simulink model "ArduCopter_3DR"  (R2016b)
settings: Solver=ode45  StartTime=0.0  StopTime=10.0  RelTol=1e-3  EnableMultiTasking=on
undefined symbols (not defined in the file): i_max, i_min, Jm, k_thrust, k_torque, L, R, v_max, v_min
settings Model: Creator=pa872d  LastModifiedBy=aaronniemiec
settings DataIOCC: LimitDataPoints=on  SaveFormat=Array
settings OptimizationCC: LifeSpan=inf
settings DebuggingCC: SFUnexpectedBacktrackingDiag=warning  SFNoUnconditionalDefaultTransitionDiag=warning  SFExecutionAtInitializationDiag=none
settings HardwareCC: ProdBitPerPointer=32  ProdBitPerSizeT=32  ProdBitPerPtrDiffT=32  ProdLargestAtomicFloat=None  ProdIntDivRoundTo=Undefined  ProdEndianess=Unspecified  ProdWordSize=32  ProdHWDeviceType=32-bit Generic
settings ModelReferenceCC: PropagateSignalLabelsOutOfModel=off
settings GRTTargetCC: TargetLangStandard=C89/C90 (ANSI)  GeneratePreprocessorConditionals=Disable all
settings ConfigComp: CovMetricSettings=dw  CovHtmlReporting=on  CovSaveCumulativeToWorkspaceVar=on  CovSaveSingleToWorkspaceVar=on  CovExternalEMLEnable=off

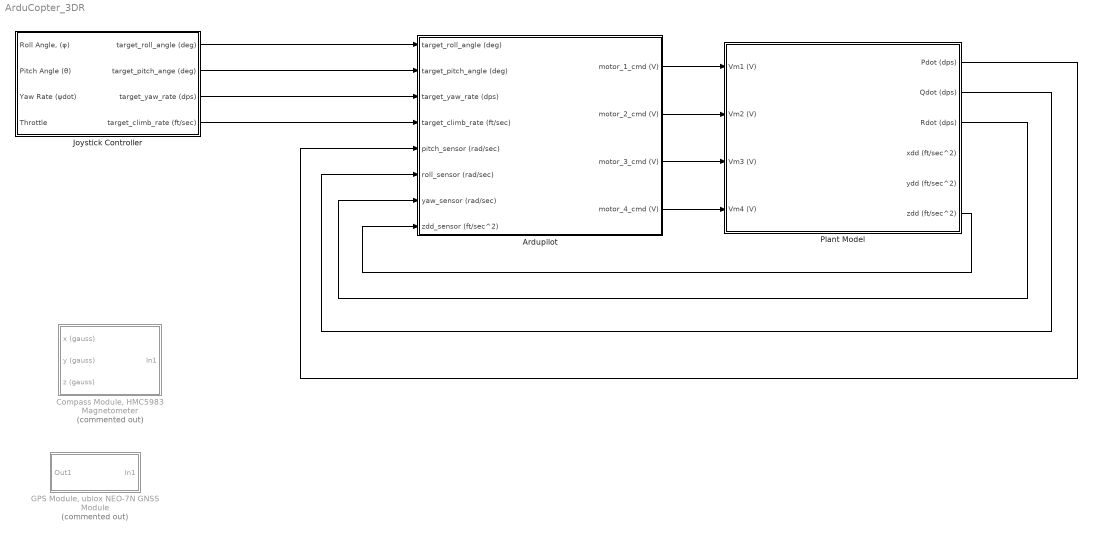
== system ArduCopter_3DR ==
  Ardupilot : Subsystem
  "Compass Module, HMC5983 Magnetometer" : Subsystem  Commented=on
  "GPS Module, ublox NEO-7N GNSS Module" : Subsystem  Commented=on
  Joystick Controller : Subsystem
  Plant Model : Subsystem
  wires:
  Joystick Controller/1(target_roll_angle (deg)) -> Ardupilot/1(target_roll_angle (deg))
  Joystick Controller/2(target_pitch_ange (deg)) -> Ardupilot/2(target_pitch_angle (deg))
  Joystick Controller/3(target_yaw_rate (dps)) -> Ardupilot/3(target_yaw_rate (dps))
  Joystick Controller/4(target_climb_rate (ft/sec)) -> Ardupilot/4(target_climb_rate (ft/sec))
  Plant Model/1(Pdot (dps)) -> Ardupilot/5(pitch_sensor (rad/sec))
  Plant Model/3(Rdot (dps)) -> Ardupilot/7(yaw_sensor (rad/sec))
  Ardupilot/1(motor_1_cmd (V)) -> Plant Model/1(Vm1 (V))
  Ardupilot/2(motor_2_cmd (V)) -> Plant Model/2(Vm2 (V))
  Ardupilot/3(motor_3_cmd (V)) -> Plant Model/3(Vm3 (V))
  Ardupilot/4(motor_4_cmd (V)) -> Plant Model/4(Vm4 (V))
  Plant Model/2(Qdot (dps)) -> Ardupilot/6(roll_sensor (rad/sec))
  Plant Model/6(zdd (ft/sec^2)) -> Ardupilot/8(zdd_sensor (ft/sec^2))

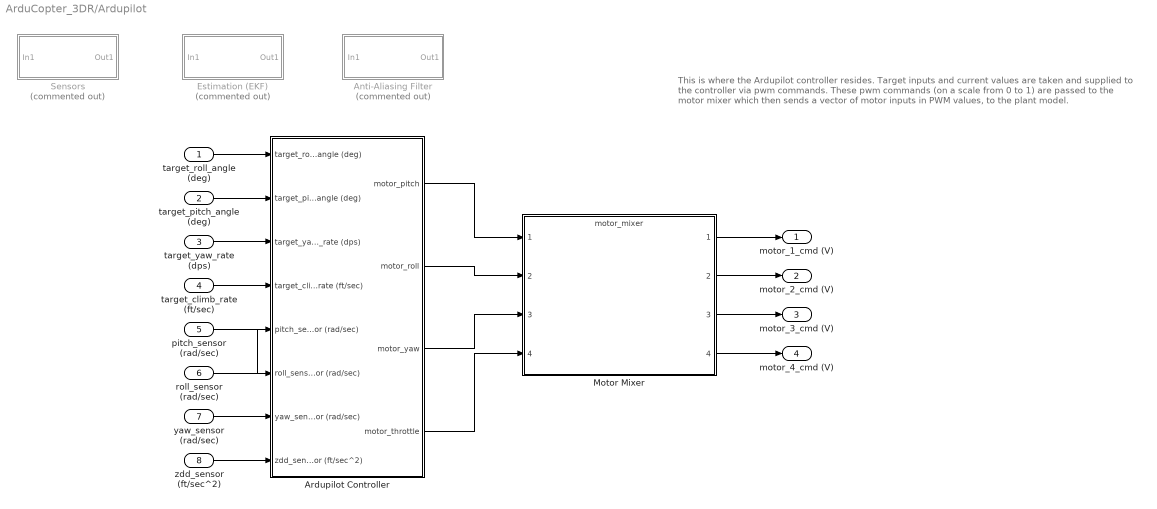
== system ArduCopter_3DR/Ardupilot ==
  note: This is where the Ardupilot controller resides. Target inputs and current values are taken and
      | supplied to the controller via pwm commands. These pwm commands (on a scale from 0 to 1) are passed to the motor mixer which then
      | sends a vector of motor inputs in PWM values, to the plant model.
  target_roll_angle (deg) : Inport
  target_pitch_angle (deg) : Inport  Port=2
  target_yaw_rate (dps) : Inport  Port=3
  target_climb_rate (ft/sec) : Inport  Port=4
  pitch_sensor (rad/sec) : Inport  Port=5
  roll_sensor (rad/sec) : Inport  Port=6
  yaw_sensor (rad/sec) : Inport  Port=7
  zdd_sensor (ft/sec^2) : Inport  Port=8
  Anti-Aliasing Filter : Subsystem  Commented=on
  Ardupilot Controller : Subsystem
  Estimation (EKF) : Subsystem  Commented=on
  Motor Mixer : ModelReference  ModelNameDialog=motor_mixer.slx  SimulationMode=Normal  ModelReferenceVersion=1.6
  Sensors : Subsystem  Commented=on
  motor_1_cmd (V) : Outport
  motor_2_cmd (V) : Outport  Port=2
  motor_3_cmd (V) : Outport  Port=3
  motor_4_cmd (V) : Outport  Port=4
  wires:
  Motor Mixer/2 -> motor_2_cmd (V)/1
  Motor Mixer/4 -> motor_4_cmd (V)/1
  Motor Mixer/3 -> motor_3_cmd (V)/1
  target_roll_angle (deg)/1 -> Ardupilot Controller/1(target_roll_angle (deg))
  target_pitch_angle (deg)/1 -> Ardupilot Controller/2(target_pitch_angle (deg))
  target_yaw_rate (dps)/1 -> Ardupilot Controller/3(target_yaw_rate (dps))
  target_climb_rate (ft/sec)/1 -> Ardupilot Controller/4(target_climb_rate (ft/sec))
  Motor Mixer/1 -> motor_1_cmd (V)/1
  yaw_sensor (rad/sec)/1 -> Ardupilot Controller/7(yaw_sensor (rad/sec))
  zdd_sensor (ft/sec^2)/1 -> Ardupilot Controller/8(zdd_sensor (ft/sec^2))
  pitch_sensor (rad/sec)/1 -> Ardupilot Controller/6(roll_sensor (rad/sec))
  roll_sensor (rad/sec)/1 -> Ardupilot Controller/5(pitch_sensor (rad/sec))
  Ardupilot Controller/1(motor_pitch) -> Motor Mixer/1
  Ardupilot Controller/2(motor_roll) -> Motor Mixer/2
  Ardupilot Controller/3(motor_yaw) -> Motor Mixer/3
  Ardupilot Controller/4(motor_throttle) -> Motor Mixer/4

== system ArduCopter_3DR/Compass Module, HMC5983 Magnetometer ==
  In1 : Inport
  x (gauss) : Outport
  y (gauss) : Outport  Port=2
  z (gauss) : Outport  Port=3

== system ArduCopter_3DR/GPS Module, ublox NEO-7N GNSS Module ==
  In1 : Inport
  Out1 : Outport
  wires:
  In1/1 -> Out1/1

== system ArduCopter_3DR/Joystick Controller ==
  "Roll Angle, (φ)" : Inport
  Pitch Angle (θ) : Inport  Port=2
  Yaw Rate (ψdot) : Inport  Port=3
  Throttle : Inport  Port=4
  target_roll_angle (deg) : Outport
  target_pitch_ange (deg) : Outport  Port=2
  target_yaw_rate (dps) : Outport  Port=3
  target_climb_rate (ft/sec) : Outport  Port=4
  wires:
  Yaw Rate (ψdot)/1 -> target_yaw_rate (dps)/1
  Throttle/1 -> target_climb_rate (ft/sec)/1
  Pitch Angle (θ)/1 -> target_pitch_ange (deg)/1
  "Roll Angle, (φ)"/1 -> target_roll_angle (deg)/1

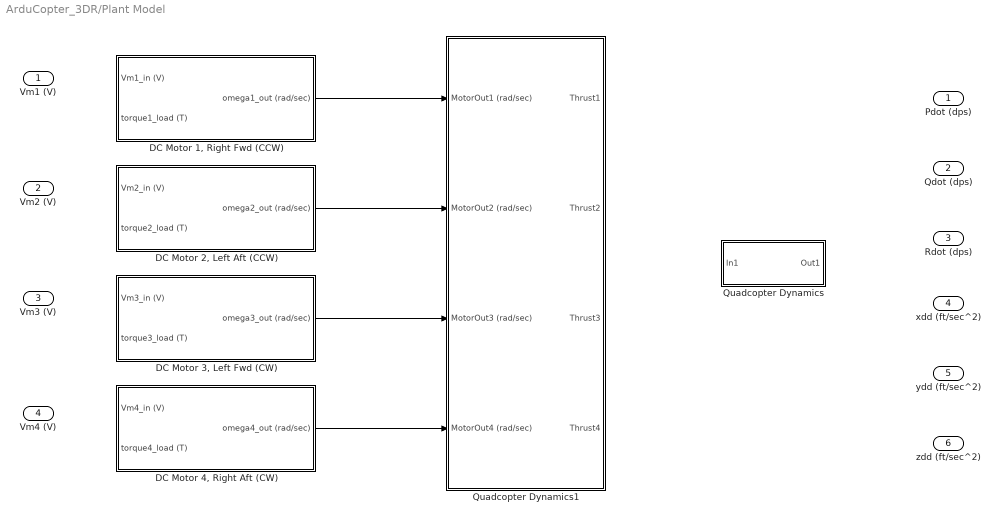
== system ArduCopter_3DR/Plant Model ==
  Vm1 (V) : Inport
  Vm2 (V) : Inport  Port=2
  Vm3 (V) : Inport  Port=3
  Vm4 (V) : Inport  Port=4
  "DC Motor 1, Right Fwd (CCW)" : Subsystem
  "DC Motor 2, Left Aft (CCW)" : Subsystem
  "DC Motor 3, Left Fwd (CW)" : Subsystem
  "DC Motor 4, Right Aft (CW)" : Subsystem
  Quadcopter Dynamics : Subsystem
  Quadcopter Dynamics1 : Subsystem
  Pdot (dps) : Outport
  Qdot (dps) : Outport  Port=2
  Rdot (dps) : Outport  Port=3
  xdd (ft/sec^2) : Outport  Port=4
  ydd (ft/sec^2) : Outport  Port=5
  zdd (ft/sec^2) : Outport  Port=6
  wires:
  "DC Motor 1, Right Fwd (CCW)"/1(omega1_out (rad/sec)) -> Quadcopter Dynamics1/1(MotorOut1 (rad/sec))
  "DC Motor 2, Left Aft (CCW)"/1(omega2_out (rad/sec)) -> Quadcopter Dynamics1/2(MotorOut2 (rad/sec))
  "DC Motor 3, Left Fwd (CW)"/1(omega3_out (rad/sec)) -> Quadcopter Dynamics1/3(MotorOut3 (rad/sec))
  "DC Motor 4, Right Aft (CW)"/1(omega4_out (rad/sec)) -> Quadcopter Dynamics1/4("MotorOut4 (rad/sec) ")

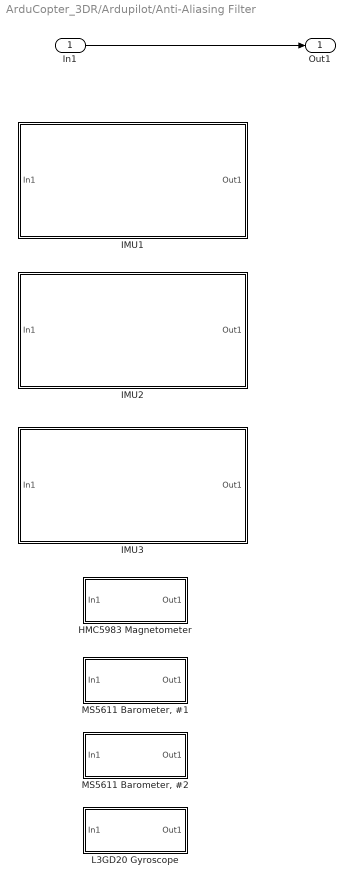
== system ArduCopter_3DR/Ardupilot/Anti-Aliasing Filter ==
  In1 : Inport
  HMC5983 Magnetometer : Subsystem
  IMU1 : Subsystem
  IMU2 : Subsystem
  IMU3 : Subsystem
  L3GD20 Gyroscope : Subsystem
  "MS5611 Barometer, #1" : Subsystem
  "MS5611 Barometer, #2" : Subsystem
  Out1 : Outport
  wires:
  In1/1 -> Out1/1

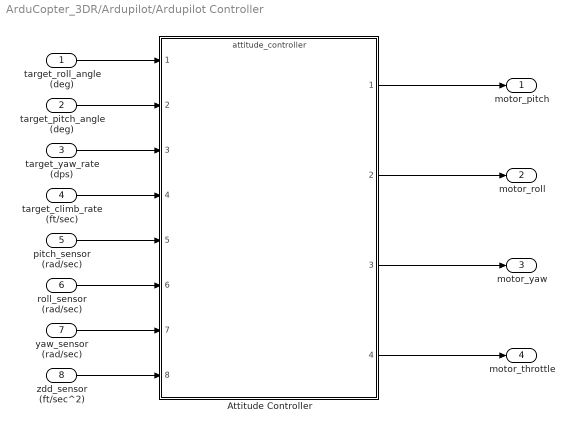
== system ArduCopter_3DR/Ardupilot/Ardupilot Controller ==
  target_roll_angle (deg) : Inport
  target_pitch_angle (deg) : Inport  Port=2
  target_yaw_rate (dps) : Inport  Port=3
  target_climb_rate (ft/sec) : Inport  Port=4
  pitch_sensor (rad/sec) : Inport  Port=5
  roll_sensor (rad/sec) : Inport  Port=6
  yaw_sensor (rad/sec) : Inport  Port=7
  zdd_sensor (ft/sec^2) : Inport  Port=8
  Attitude Controller : ModelReference  ModelNameDialog=attitude_controller.slx  SimulationMode=Normal  ModelReferenceVersion=1.15
  motor_pitch : Outport
  motor_roll : Outport  Port=2
  motor_yaw : Outport  Port=3
  motor_throttle : Outport  Port=4
  wires:
  Attitude Controller/4 -> motor_throttle/1
  Attitude Controller/3 -> motor_yaw/1
  target_roll_angle (deg)/1 -> Attitude Controller/1
  target_pitch_angle (deg)/1 -> Attitude Controller/2
  target_yaw_rate (dps)/1 -> Attitude Controller/3
  target_climb_rate (ft/sec)/1 -> Attitude Controller/4
  yaw_sensor (rad/sec)/1 -> Attitude Controller/7
  zdd_sensor (ft/sec^2)/1 -> Attitude Controller/8
  roll_sensor (rad/sec)/1 -> Attitude Controller/6
  pitch_sensor (rad/sec)/1 -> Attitude Controller/5
  Attitude Controller/2 -> motor_roll/1
  Attitude Controller/1 -> motor_pitch/1

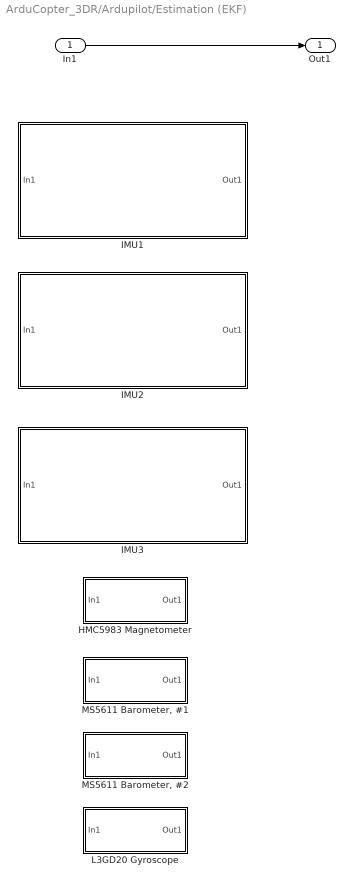
== system ArduCopter_3DR/Ardupilot/Estimation (EKF) ==
  In1 : Inport
  HMC5983 Magnetometer : Subsystem
  IMU1 : Subsystem
  IMU2 : Subsystem
  IMU3 : Subsystem
  L3GD20 Gyroscope : Subsystem
  "MS5611 Barometer, #1" : Subsystem
  "MS5611 Barometer, #2" : Subsystem
  Out1 : Outport
  wires:
  In1/1 -> Out1/1

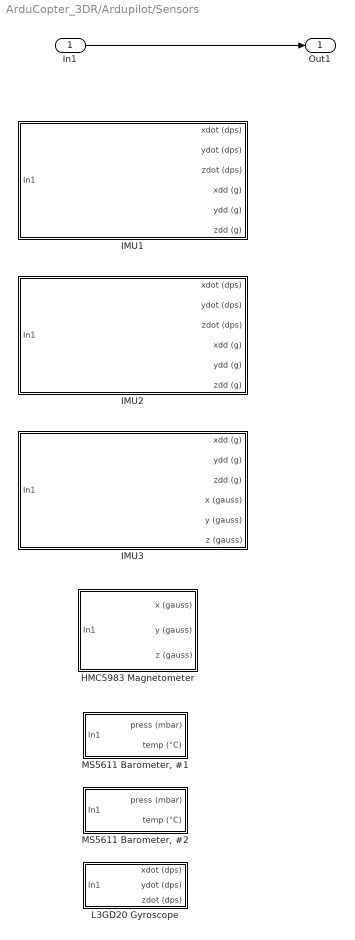
== system ArduCopter_3DR/Ardupilot/Sensors ==
  In1 : Inport
  HMC5983 Magnetometer : Subsystem
  IMU1 : Subsystem
  IMU2 : Subsystem
  IMU3 : Subsystem
  L3GD20 Gyroscope : Subsystem
  "MS5611 Barometer, #1" : Subsystem
  "MS5611 Barometer, #2" : Subsystem
  Out1 : Outport
  wires:
  In1/1 -> Out1/1

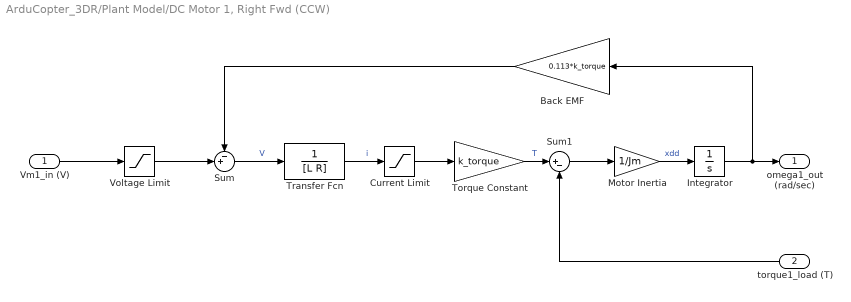
== system ArduCopter_3DR/Plant Model/DC Motor 1, Right Fwd (CCW) ==
  Vm1_in (V) : Inport
  torque1_load (T) : Inport  Port=2
  Back EMF : Gain  Gain=0.113*k_torque
  Current Limit : Saturate  UpperLimit=i_max  LowerLimit=i_min
  Integrator : Integrator
  Motor Inertia : Gain  Gain=1/Jm
  Sum : Sum  Inputs=-+|
  Sum1 : Sum  Inputs=|+-
  Torque Constant : Gain  Gain=k_torque
  Transfer Fcn : TransferFcn  Denominator=[L R]
  Voltage Limit : Saturate  UpperLimit=v_max  LowerLimit=v_min
  omega1_out (rad/sec) : Outport
  wires:
  Vm1_in (V)/1 -> Voltage Limit/1
  Voltage Limit/1 -> Sum/2
  torque1_load (T)/1 -> Sum1/2
  Sum1/1 -> Motor Inertia/1
  Integrator/1 -> omega1_out (rad/sec)/1, Back EMF/1
  Motor Inertia/1 -> Integrator/1  "xdd"
  Back EMF/1 -> Sum/1
  Torque Constant/1 -> Sum1/1  "T"
  Current Limit/1 -> Torque Constant/1
  Sum/1 -> Transfer Fcn/1  "V"
  Transfer Fcn/1 -> Current Limit/1  "i"

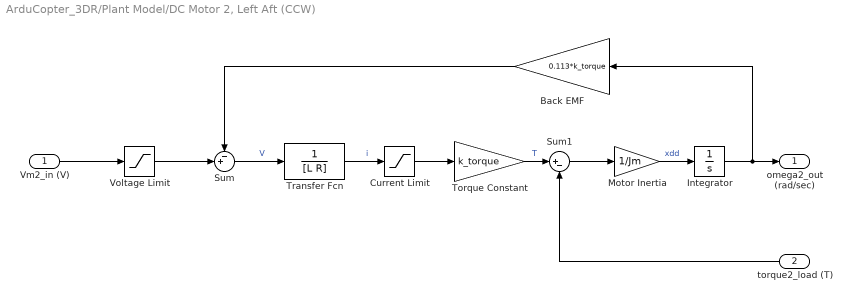
== system ArduCopter_3DR/Plant Model/DC Motor 2, Left Aft (CCW) ==
  Vm2_in (V) : Inport
  torque2_load (T) : Inport  Port=2
  Back EMF : Gain  Gain=0.113*k_torque
  Current Limit : Saturate  UpperLimit=i_max  LowerLimit=i_min
  Integrator : Integrator
  Motor Inertia : Gain  Gain=1/Jm
  Sum : Sum  Inputs=-+|
  Sum1 : Sum  Inputs=|+-
  Torque Constant : Gain  Gain=k_torque
  Transfer Fcn : TransferFcn  Denominator=[L R]
  Voltage Limit : Saturate  UpperLimit=v_max  LowerLimit=v_min
  omega2_out (rad/sec) : Outport
  wires:
  Vm2_in (V)/1 -> Voltage Limit/1
  Voltage Limit/1 -> Sum/2
  torque2_load (T)/1 -> Sum1/2
  Sum1/1 -> Motor Inertia/1
  Integrator/1 -> omega2_out (rad/sec)/1, Back EMF/1
  Motor Inertia/1 -> Integrator/1  "xdd"
  Back EMF/1 -> Sum/1
  Torque Constant/1 -> Sum1/1  "T"
  Current Limit/1 -> Torque Constant/1
  Sum/1 -> Transfer Fcn/1  "V"
  Transfer Fcn/1 -> Current Limit/1  "i"

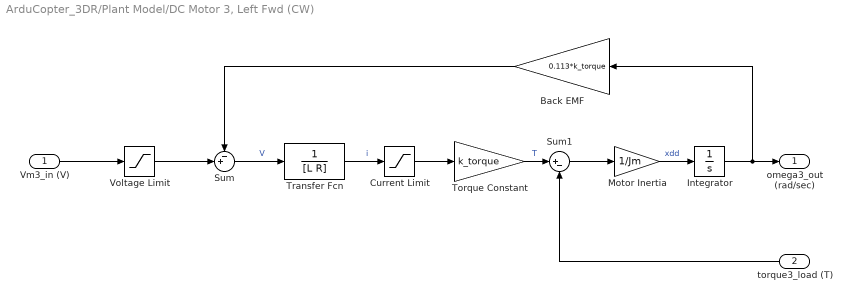
== system ArduCopter_3DR/Plant Model/DC Motor 3, Left Fwd (CW) ==
  Vm3_in (V) : Inport
  torque3_load (T) : Inport  Port=2
  Back EMF : Gain  Gain=0.113*k_torque
  Current Limit : Saturate  UpperLimit=i_max  LowerLimit=i_min
  Integrator : Integrator
  Motor Inertia : Gain  Gain=1/Jm
  Sum : Sum  Inputs=-+|
  Sum1 : Sum  Inputs=|+-
  Torque Constant : Gain  Gain=k_torque
  Transfer Fcn : TransferFcn  Denominator=[L R]
  Voltage Limit : Saturate  UpperLimit=v_max  LowerLimit=v_min
  omega3_out (rad/sec) : Outport
  wires:
  Vm3_in (V)/1 -> Voltage Limit/1
  Voltage Limit/1 -> Sum/2
  torque3_load (T)/1 -> Sum1/2
  Sum1/1 -> Motor Inertia/1
  Integrator/1 -> omega3_out (rad/sec)/1, Back EMF/1
  Motor Inertia/1 -> Integrator/1  "xdd"
  Back EMF/1 -> Sum/1
  Torque Constant/1 -> Sum1/1  "T"
  Current Limit/1 -> Torque Constant/1
  Sum/1 -> Transfer Fcn/1  "V"
  Transfer Fcn/1 -> Current Limit/1  "i"

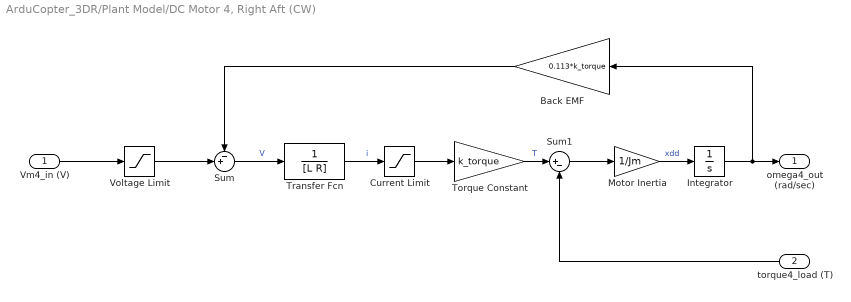
== system ArduCopter_3DR/Plant Model/DC Motor 4, Right Aft (CW) ==
  Vm4_in (V) : Inport
  torque4_load (T) : Inport  Port=2
  Back EMF : Gain  Gain=0.113*k_torque
  Current Limit : Saturate  UpperLimit=i_max  LowerLimit=i_min
  Integrator : Integrator
  Motor Inertia : Gain  Gain=1/Jm
  Sum : Sum  Inputs=-+|
  Sum1 : Sum  Inputs=|+-
  Torque Constant : Gain  Gain=k_torque
  Transfer Fcn : TransferFcn  Denominator=[L R]
  Voltage Limit : Saturate  UpperLimit=v_max  LowerLimit=v_min
  omega4_out (rad/sec) : Outport
  wires:
  Vm4_in (V)/1 -> Voltage Limit/1
  Voltage Limit/1 -> Sum/2
  torque4_load (T)/1 -> Sum1/2
  Sum1/1 -> Motor Inertia/1
  Integrator/1 -> omega4_out (rad/sec)/1, Back EMF/1
  Motor Inertia/1 -> Integrator/1  "xdd"
  Back EMF/1 -> Sum/1
  Torque Constant/1 -> Sum1/1  "T"
  Current Limit/1 -> Torque Constant/1
  Sum/1 -> Transfer Fcn/1  "V"
  Transfer Fcn/1 -> Current Limit/1  "i"

== system ArduCopter_3DR/Plant Model/Quadcopter Dynamics ==
  In1 : Inport
  Out1 : Outport
  wires:
  In1/1 -> Out1/1

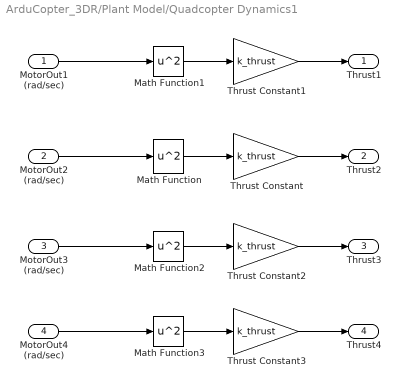
== system ArduCopter_3DR/Plant Model/Quadcopter Dynamics1 ==
  MotorOut1 (rad/sec) : Inport
  MotorOut2 (rad/sec) : Inport  Port=2
  MotorOut3 (rad/sec) : Inport  Port=3
  "MotorOut4 (rad/sec) " : Inport  Port=4
  Math Function{,1..3} (4 alike) : Math  Operator=square  SaturateOnIntegerOverflow=on
  Thrust Constant{,1..3} (4 alike) : Gain  Gain=k_thrust
  Thrust1 : Outport
  Thrust2 : Outport  Port=2
  Thrust3 : Outport  Port=3
  Thrust4 : Outport  Port=4
  wires:
  MotorOut2 (rad/sec)/1 -> Math Function/1
  Math Function/1 -> Thrust Constant/1
  Thrust Constant/1 -> Thrust2/1
  MotorOut1 (rad/sec)/1 -> Math Function1/1
  Math Function1/1 -> Thrust Constant1/1
  Thrust Constant1/1 -> Thrust1/1
  MotorOut3 (rad/sec)/1 -> Math Function2/1
  Math Function2/1 -> Thrust Constant2/1
  Thrust Constant2/1 -> Thrust3/1
  "MotorOut4 (rad/sec) "/1 -> Math Function3/1
  Math Function3/1 -> Thrust Constant3/1
  Thrust Constant3/1 -> Thrust4/1

== system ArduCopter_3DR/Ardupilot/Anti-Aliasing Filter/HMC5983 Magnetometer ==
  In1 : Inport
  Out1 : Outport
  wires:
  In1/1 -> Out1/1

== system ArduCopter_3DR/Ardupilot/Anti-Aliasing Filter/IMU1 ==
  In1 : Inport
  MPU6000 Accelerometer : Subsystem
  MPU6000 Gyroscope : Subsystem
  Out1 : Outport
  wires:
  In1/1 -> Out1/1

== system ArduCopter_3DR/Ardupilot/Anti-Aliasing Filter/IMU2 ==
  In1 : Inport
  MPU6000 Accelerometer : Subsystem
  MPU6000 Gyroscope : Subsystem
  Out1 : Outport
  wires:
  In1/1 -> Out1/1

== system ArduCopter_3DR/Ardupilot/Anti-Aliasing Filter/IMU3 ==
  In1 : Inport
  LSM303D Accelerometer : Subsystem
  LSM303D Magnetometer : Subsystem
  Out1 : Outport
  wires:
  In1/1 -> Out1/1

== system ArduCopter_3DR/Ardupilot/Anti-Aliasing Filter/L3GD20 Gyroscope ==
  In1 : Inport
  Out1 : Outport
  wires:
  In1/1 -> Out1/1

== system ArduCopter_3DR/Ardupilot/Anti-Aliasing Filter/MS5611 Barometer, #1 ==
  In1 : Inport
  Out1 : Outport
  wires:
  In1/1 -> Out1/1

== system ArduCopter_3DR/Ardupilot/Anti-Aliasing Filter/MS5611 Barometer, #2 ==
  In1 : Inport
  Out1 : Outport
  wires:
  In1/1 -> Out1/1

== system ArduCopter_3DR/Ardupilot/Estimation (EKF)/HMC5983 Magnetometer ==
  In1 : Inport
  Out1 : Outport
  wires:
  In1/1 -> Out1/1

== system ArduCopter_3DR/Ardupilot/Estimation (EKF)/IMU1 ==
  In1 : Inport
  MPU6000 Accelerometer : Subsystem
  MPU6000 Gyroscope : Subsystem
  Out1 : Outport
  wires:
  In1/1 -> Out1/1

== system ArduCopter_3DR/Ardupilot/Estimation (EKF)/IMU2 ==
  In1 : Inport
  MPU6000 Accelerometer : Subsystem
  MPU6000 Gyroscope : Subsystem
  Out1 : Outport
  wires:
  In1/1 -> Out1/1

== system ArduCopter_3DR/Ardupilot/Estimation (EKF)/IMU3 ==
  In1 : Inport
  LSM303D Accelerometer : Subsystem
  LSM303D Magnetometer : Subsystem
  Out1 : Outport
  wires:
  In1/1 -> Out1/1

== system ArduCopter_3DR/Ardupilot/Estimation (EKF)/L3GD20 Gyroscope ==
  In1 : Inport
  Out1 : Outport
  wires:
  In1/1 -> Out1/1

== system ArduCopter_3DR/Ardupilot/Estimation (EKF)/MS5611 Barometer, #1 ==
  In1 : Inport
  Out1 : Outport
  wires:
  In1/1 -> Out1/1

== system ArduCopter_3DR/Ardupilot/Estimation (EKF)/MS5611 Barometer, #2 ==
  In1 : Inport
  Out1 : Outport
  wires:
  In1/1 -> Out1/1

== system ArduCopter_3DR/Ardupilot/Sensors/HMC5983 Magnetometer ==
  In1 : Inport
  x (gauss) : Outport
  y (gauss) : Outport  Port=2
  z (gauss) : Outport  Port=3

== system ArduCopter_3DR/Ardupilot/Sensors/IMU1 ==
  In1 : Inport
  MPU6000 Accelerometer : Subsystem
  MPU6000 Gyroscope : Subsystem
  xdot (dps) : Outport
  ydot (dps) : Outport  Port=2
  zdot (dps) : Outport  Port=3
  xdd (g) : Outport  Port=4
  ydd (g) : Outport  Port=5
  zdd (g) : Outport  Port=6

== system ArduCopter_3DR/Ardupilot/Sensors/IMU2 ==
  In1 : Inport
  MPU6000 Accelerometer : Subsystem
  MPU6000 Gyroscope : Subsystem
  xdot (dps) : Outport
  ydot (dps) : Outport  Port=2
  zdot (dps) : Outport  Port=3
  xdd (g) : Outport  Port=4
  ydd (g) : Outport  Port=5
  zdd (g) : Outport  Port=6

== system ArduCopter_3DR/Ardupilot/Sensors/IMU3 ==
  In1 : Inport
  LSM303D Accelerometer : Subsystem
  LSM303D Magnetometer : Subsystem
  xdd (g) : Outport
  ydd (g) : Outport  Port=2
  zdd (g) : Outport  Port=3
  x (gauss) : Outport  Port=4
  y (gauss) : Outport  Port=5
  z (gauss) : Outport  Port=6

== system ArduCopter_3DR/Ardupilot/Sensors/L3GD20 Gyroscope ==
  In1 : Inport
  xdot (dps) : Outport
  ydot (dps) : Outport  Port=2
  zdot (dps) : Outport  Port=3

== system ArduCopter_3DR/Ardupilot/Sensors/MS5611 Barometer, #1 ==
  In1 : Inport
  press (mbar) : Outport
  temp (°C) : Outport  Port=2

== system ArduCopter_3DR/Ardupilot/Sensors/MS5611 Barometer, #2 ==
  In1 : Inport
  press (mbar) : Outport
  temp (°C) : Outport  Port=2

== system ArduCopter_3DR/Ardupilot/Anti-Aliasing Filter/IMU1/MPU6000 Accelerometer ==
  In1 : Inport
  Out1 : Outport
  wires:
  In1/1 -> Out1/1

== system ArduCopter_3DR/Ardupilot/Anti-Aliasing Filter/IMU1/MPU6000 Gyroscope ==
  In1 : Inport
  Out1 : Outport
  wires:
  In1/1 -> Out1/1

== system ArduCopter_3DR/Ardupilot/Anti-Aliasing Filter/IMU2/MPU6000 Accelerometer ==
  In1 : Inport
  Out1 : Outport
  wires:
  In1/1 -> Out1/1

== system ArduCopter_3DR/Ardupilot/Anti-Aliasing Filter/IMU2/MPU6000 Gyroscope ==
  In1 : Inport
  Out1 : Outport
  wires:
  In1/1 -> Out1/1

== system ArduCopter_3DR/Ardupilot/Anti-Aliasing Filter/IMU3/LSM303D Accelerometer ==
  In1 : Inport
  Out1 : Outport
  wires:
  In1/1 -> Out1/1

== system ArduCopter_3DR/Ardupilot/Anti-Aliasing Filter/IMU3/LSM303D Magnetometer ==
  In1 : Inport
  Out1 : Outport
  wires:
  In1/1 -> Out1/1

== system ArduCopter_3DR/Ardupilot/Estimation (EKF)/IMU1/MPU6000 Accelerometer ==
  In1 : Inport
  Out1 : Outport
  wires:
  In1/1 -> Out1/1

== system ArduCopter_3DR/Ardupilot/Estimation (EKF)/IMU1/MPU6000 Gyroscope ==
  In1 : Inport
  Out1 : Outport
  wires:
  In1/1 -> Out1/1

== system ArduCopter_3DR/Ardupilot/Estimation (EKF)/IMU2/MPU6000 Accelerometer ==
  In1 : Inport
  Out1 : Outport
  wires:
  In1/1 -> Out1/1

== system ArduCopter_3DR/Ardupilot/Estimation (EKF)/IMU2/MPU6000 Gyroscope ==
  In1 : Inport
  Out1 : Outport
  wires:
  In1/1 -> Out1/1

== system ArduCopter_3DR/Ardupilot/Estimation (EKF)/IMU3/LSM303D Accelerometer ==
  In1 : Inport
  Out1 : Outport
  wires:
  In1/1 -> Out1/1

== system ArduCopter_3DR/Ardupilot/Estimation (EKF)/IMU3/LSM303D Magnetometer ==
  In1 : Inport
  Out1 : Outport
  wires:
  In1/1 -> Out1/1

== system ArduCopter_3DR/Ardupilot/Sensors/IMU1/MPU6000 Accelerometer ==
  In1 : Inport
  xdd (g) : Outport
  ydd (g) : Outport  Port=2
  zdd (g) : Outport  Port=3

== system ArduCopter_3DR/Ardupilot/Sensors/IMU1/MPU6000 Gyroscope ==
  In1 : Inport
  xdot (dps) : Outport
  ydot (dps) : Outport  Port=2
  zdot (dps) : Outport  Port=3

== system ArduCopter_3DR/Ardupilot/Sensors/IMU2/MPU6000 Accelerometer ==
  In1 : Inport
  xdd (g) : Outport
  ydd (g) : Outport  Port=2
  zdd (g) : Outport  Port=3

== system ArduCopter_3DR/Ardupilot/Sensors/IMU2/MPU6000 Gyroscope ==
  In1 : Inport
  xdot (dps) : Outport
  ydot (dps) : Outport  Port=2
  zdot (dps) : Outport  Port=3

== system ArduCopter_3DR/Ardupilot/Sensors/IMU3/LSM303D Accelerometer ==
  In1 : Inport
  xdd (g) : Outport
  ydd (g) : Outport  Port=2
  zdd (g) : Outport  Port=3

== system ArduCopter_3DR/Ardupilot/Sensors/IMU3/LSM303D Magnetometer ==
  In1 : Inport
  x (gauss) : Outport
  y (gauss) : Outport  Port=2
  z (gauss) : Outport  Port=3
